simulink model "Complete_ballsegway_model"  (R2024b)
settings: Solver=VariableStepAuto  StartTime=0.0  StopTime=10  RelTol=1e-3
settings Model: Creator=sumit  LastModifiedBy=yugan
settings DebuggingCC: AlgebraicLoopMsg=none

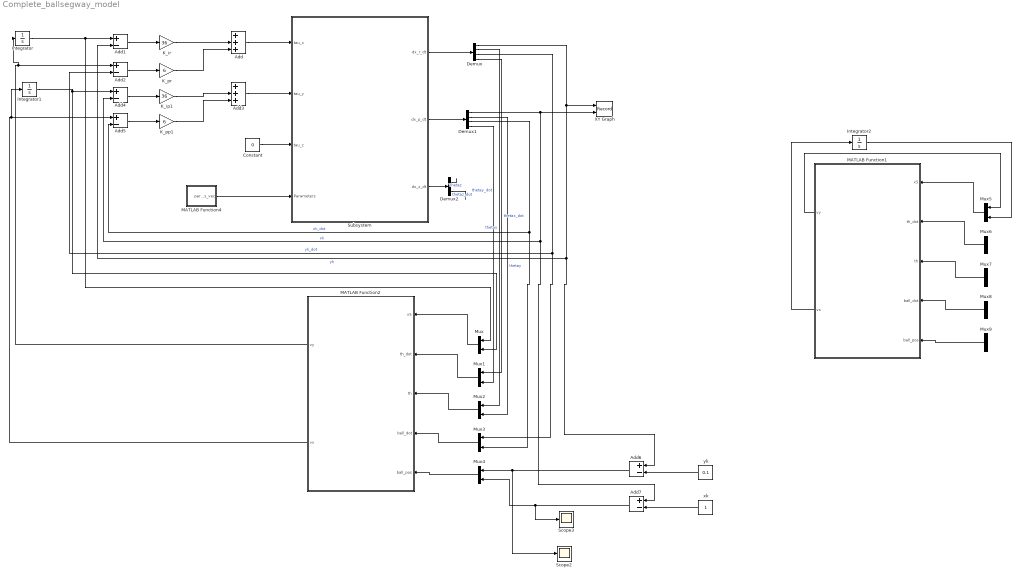
== system Complete_ballsegway_model ==
  Add : Sum  Inputs=+++
  Add{1..2,4..7} (6 alike) : Sum  Inputs=+-
  Add3 : Sum  Inputs=+++
  Constant : Constant  Value=0
  Demux : Demux
  Demux1 : Demux
  Demux2 : Demux  Outputs=2
  Integrator : Integrator
  Integrator1 : Integrator
  Integrator2 : Integrator
  K_ip1 : Gain  Gain=36
  K_ir : Gain  Gain=36
  K_pp1 : Gain  Gain=6
  K_pr : Gain  Gain=6
  MATLAB Function1 : MATLAB Function  TreatAsAtomicUnit=on
  MATLAB Function2 : MATLAB Function  TreatAsAtomicUnit=on
  MATLAB Function4 : MATLAB Function  TreatAsAtomicUnit=on
  Mux{,1..9} (10 alike) : Mux  Inputs=2
  Scope2 : Scope
  Scope3 : Scope
  Subsystem : Subsystem
  XY Graph : Record  FileSettingsInternal="{\"entries\":[{\"content\":{\"excelSettings\":{\"content\":{},\"type\":\"Streamout.ExcelSettings\"}},\"type\":\"Streamout.FileSettingStorage\",\"uuid\":\"\"}],\"packageUris\":[\"http:\\/\\/schema.mathworks.com\\/mf0\\/streamout_blocks\\/R2020a\"],\"version\":\"1.0\"}"  Layout=[1 1]  SignalsInternal="{\"entries\":[{\"content\":{\"signals\":[{\"content\":{\"blockPath\":[],\"dimensions\":[1,1],\"domain\":\"\",\"lineColor\":\"#a2142f\",\"plots\":[ 1 ],\"port\":1,\"signalID\":1,\"signalName\":\"yk\"},\"type\":\"RecordBlkView.Signal\",\"uuid\":\"\"},{\"content\":{\"blockPath\":[],\"dimensions\":[1,1],\"domain\":\"\",\"lineColor\":\"#139fff\",\"plots\":[ 1 ],\"port\":2,\"signalID\":2,\"signalName\":\"xk\"},\"type\":\"RecordBlkView.Signal\",\"uuid\":\"\"}]},\"type\":\"RecordBlkView.InputSignals\",\"uuid\":\"\"}],\"packageUris\":[\"http:\\/\\/schema.mathworks.com\\/mf0\\/streamout_blocks\\/R2020a\"],\"version\":\"1.0\"}"  VisualizationBindings="{\"xyplotplugin\":{\"info\":[{\"series\":[{\"bindingParametersList\":[{\"parameter\":\"Y-Axis\",\"signalID\":1,\"signalName\":\"yk\"}],\"seriesID\":0}],\"subplotID\":1}]}}"  CompatibilityTag=XY
  xk : Constant
  yk : Constant  Value=0.1
  wires:
  Subsystem/3(dx_z_dt) -> Demux2/1
  MATLAB Function4/1(params_vec) -> Subsystem/4(Parameters)
  Mux/1 -> MATLAB Function2/1(x5)
  Integrator1/1 -> Mux/2, Add4/1
  Add/1 -> Subsystem/1(tau_x)
  K_ir/1 -> Add/2
  Add1/1 -> K_ir/1
  Subsystem/1(dx_r_dt) -> Demux/1
  Subsystem/2(dx_p_dt) -> Demux1/1
  Demux/1 -> Add1/2, Add6/1, XY Graph/1  "yk"
  Demux/2 -> Mux2/1  "thetax"
  Demux/3 -> Mux3/1, Add2/2  "yk_dot"
  Demux/4 -> Mux1/1  "thetax_dot"
  Demux1/2 -> Mux2/2  "thetay"
  Demux1/3 -> Mux3/2, Add5/2  "xk_dot"
  Demux1/4 -> Mux1/2  "thetay_dot"
  Demux2/1 -> ?  "Thetaz"
  Demux2/2 -> ?  "thetaz_dot"
  Integrator/1 -> Mux/1, Add1/1
  K_pr/1 -> Add/3
  Add2/1 -> K_pr/1
  Demux1/1 -> Add7/1, Add4/2, XY Graph/2  "xk"
  Add4/1 -> K_ip1/1
  K_pp1/1 -> Add3/3
  K_ip1/1 -> Add3/2
  Add3/1 -> Subsystem/2(tau_y)
  Add5/1 -> K_pp1/1
  Constant/1 -> Subsystem/3(tau_z)
  Mux1/1 -> MATLAB Function2/2(th_dot)
  Mux2/1 -> MATLAB Function2/3(th)
  Mux3/1 -> MATLAB Function2/4(ball_dot)
  Mux4/1 -> MATLAB Function2/5(ball_pos)
  Add6/1 -> Scope2/1, Mux4/1
  yk/1 -> Add6/2
  Add7/1 -> Scope3/1, Mux4/2
  xk/1 -> Add7/2
  MATLAB Function2/1(vy) -> Add2/1, Integrator/1
  MATLAB Function2/2(vx) -> Add5/1, Integrator1/1
  MATLAB Function1/1(vy) -> Mux5/1
  Mux5/1 -> MATLAB Function1/1(x5)
  Mux7/1 -> MATLAB Function1/3(th)
  Mux8/1 -> MATLAB Function1/4(ball_dot)
  Mux6/1 -> MATLAB Function1/2(th_dot)
  Mux9/1 -> MATLAB Function1/5(ball_pos)
  MATLAB Function1/2(vx) -> Integrator2/1
  ? -> Mux6/1
  ? -> Mux6/2
  ? -> Mux7/1
  ? -> Mux7/2
  ? -> Mux8/1
  ? -> Mux8/2
  ? -> Mux9/1
  ? -> Mux9/2
  Integrator2/1 -> Mux5/2

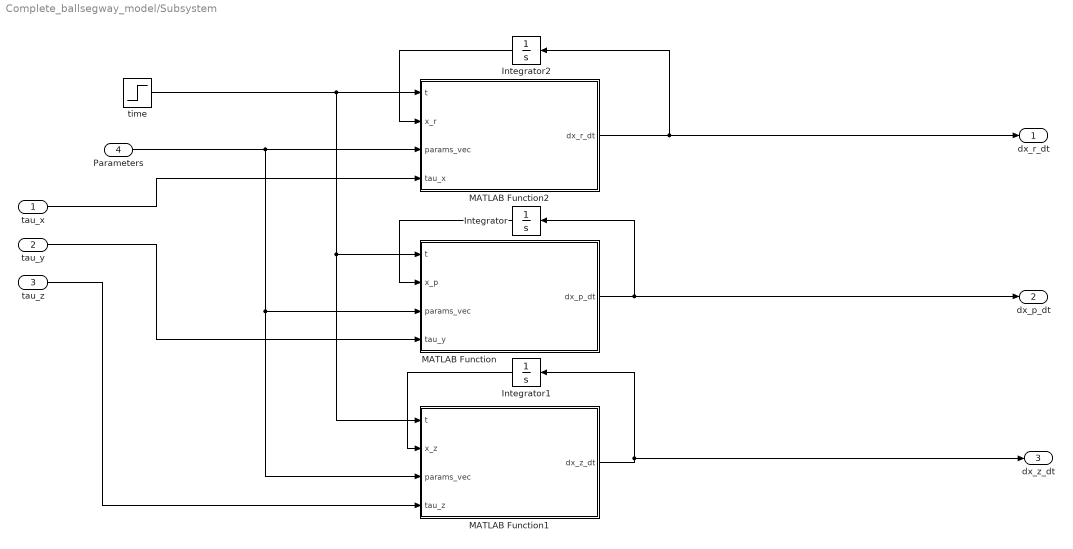
== system Complete_ballsegway_model/Subsystem ==
  tau_x : Inport
  tau_y : Inport  Port=2
  tau_z : Inport  Port=3
  Parameters : Inport  Port=4
  Integrator : Integrator  InitialCondition=[0; 0; 0; 0]
  Integrator1 : Integrator  InitialCondition=[0 ;0]
  Integrator2 : Integrator  InitialCondition=[0; 0; 0; 0]
  MATLAB Function : MATLAB Function  TreatAsAtomicUnit=on
  MATLAB Function1 : MATLAB Function  TreatAsAtomicUnit=on
  MATLAB Function2 : MATLAB Function  TreatAsAtomicUnit=on
  time : Step  After=10  SampleTime=0
  dx_r_dt : Outport
  dx_p_dt : Outport  Port=2
  dx_z_dt : Outport  Port=3
  wires:
  time/1 -> MATLAB Function1/1(t), MATLAB Function/1(t), MATLAB Function2/1(t)
  Integrator1/1 -> MATLAB Function1/2(x_z)
  Parameters/1 -> MATLAB Function/3(params_vec), MATLAB Function1/3(params_vec), MATLAB Function2/3(params_vec)
  Integrator2/1 -> MATLAB Function2/2(x_r)
  MATLAB Function1/1(dx_z_dt) -> Integrator1/1, dx_z_dt/1
  tau_z/1 -> MATLAB Function1/4(tau_z)
  Integrator/1 -> MATLAB Function/2(x_p)
  tau_y/1 -> MATLAB Function/4(tau_y)
  tau_x/1 -> MATLAB Function2/4(tau_x)
  MATLAB Function/1(dx_p_dt) -> Integrator/1, dx_p_dt/1
  MATLAB Function2/1(dx_r_dt) -> dx_r_dt/1, Integrator2/1

== matlab function Complete_ballsegway_model/Subsystem/MATLAB Function1 ==
  data: t input; dx_z_dt output; x_z input; params_vec input; tau_z input
function dx_z_dt = yaw_dynamics(t, x_z, params_vec, tau_z)
% yaw_dynamics.m
%
% 1-DOF yaw dynamic model for Ball Segway.
%
% State x_z = [theta_z ; theta_z_dot]
% params_vec = 20×1 numeric parameter vector (from init_params)
% Output dx_z_dt = state derivative (2×1)

%% ---------------------------------------------------------
% Unpack Parameters From Vector
%% ---------------------------------------------------------

mk  = params_vec(1);     %#ok<NASGU> (not used)
Ik  = params_vec(2);
ma  = params_vec(3);     %#ok<NASGU>
Ix  = params_vec(4);     %#ok<NASGU>
Iy  = params_vec(5);
Iz  = params_vec(6);
l   = params_vec(7);     %#ok<NASGU>
alpha_rad = params_vec(8);
rk  = params_vec(9);
rw  = params_vec(10);
bx  = params_vec(11);    %#ok<NASGU>
dx  = params_vec(12);    %#ok<NASGU>
by  = params_vec(13);    %#ok<NASGU>
dy  = params_vec(14);    %#ok<NASGU>
bry = params_vec(15);    %#ok<NASGU>
dry = params_vec(16);    %#ok<NASGU>
brx = params_vec(17);    %#ok<NASGU>
drx = params_vec(18);    %#ok<NASGU>
g   = params_vec(19);    %#ok<NASGU>
k_motor = params_vec(20); %#ok<NASGU>

% Keep notation same as your original code
I_k_param = Ik;
I_w = Iy;


%% ---------------------------------------------------------
% Extract States
%% ---------------------------------------------------------

theta_z     = x_z(1);
theta_z_dot = x_z(2);


%% ---------------------------------------------------------
% Yaw Dynamics (Eq. 13)
%% ---------------------------------------------------------

num = I_k_param * (rk / rw) * tau_z;

den = I_k_param * Iz + ...
      3 * (I_k_param + Iz) * I_w * (rk / rw)^2 * sin(alpha_rad)^2;

theta_z_ddot = num / den;


%% ---------------------------------------------------------
% Return Derivative
%% ---------------------------------------------------------

dx_z_dt = [ theta_z_dot ;
            theta_z_ddot ];

end

== matlab function Complete_ballsegway_model/Subsystem/MATLAB Function ==
  data: t input; dx_p_dt output; x_p input; params_vec input; tau_y input
function dx_p_dt = pitch_dynamics(t, x_p, params_vec, tau_y)
% pitch_dynamics.m
%
% 2-DOF dynamic model in the X–Z plane (pitch plane).
%
% State x_p = [x_k ; theta_y ; x_k_dot ; theta_y_dot]
% params_vec = 20×1 vector from init_params()
% Output dx_p_dt = state derivative (4×1)

%% ---------------------------------------------------------
% Unpack Parameters from Vector
%% ---------------------------------------------------------

mk  = params_vec(1);     % ball mass
Ik  = params_vec(2);     % ball inertia
ma  = params_vec(3);     % body mass
Ix  = params_vec(4);     % inertia about x
Iy  = params_vec(5);     % inertia about y
Iz  = params_vec(6);     % inertia about z
l   = params_vec(7);     % COM height
alpha_rad = params_vec(8); % zenith angle
rk  = params_vec(9);     % ball radius
rw  = params_vec(10);    % omniwheel radius
bx  = params_vec(11);
dx  = params_vec(12);
by  = params_vec(13);
dy  = params_vec(14);
bry = params_vec(15);
dry = params_vec(16);
brx = params_vec(17);
drx = params_vec(18);
g   = params_vec(19);    % gravity
k_motor = params_vec(20);

% Keep original notation
I_k_param = Ik;
I_w = Iy;    % consistent with roll dynamics formulation


%% ---------------------------------------------------------
% Extract State Variables
%% ---------------------------------------------------------

x_k         = x_p(1);
theta_y     = x_p(2);
x_k_dot     = x_p(3);
theta_y_dot = x_p(4);

q_y_dot = [x_k_dot ; theta_y_dot];


%% ---------------------------------------------------------
% Mass Matrix M(q)   (Eq. 8)
%% ---------------------------------------------------------

M11 = mk + (I_k_param / rk^2) + ma + ...
      (3*I_w*cos(alpha_rad)^2) / (2*rw^2);

M12 =   ma*l*cos(theta_y) ...
      - (3*I_w*cos(alpha_rad)^2)/(2*rw^2) * rk;

M21 = M12;

M22 = ma*l^2 + ...
      (3*I_w*rk^2*cos(alpha_rad)^2)/(2*rw^2) + Iy;

M_y = [M11 M12; M21 M22];


%% ---------------------------------------------------------
% Coriolis–Centrifugal Vector
%% ---------------------------------------------------------

C_y = [ 0                            -ma*l*theta_y_dot*sin(theta_y);
        0                             0 ];


%% ---------------------------------------------------------
% Gravity Vector
%% ---------------------------------------------------------

G_y = [0;
       -ma*g*l*sin(theta_y)];


%% ---------------------------------------------------------
% Friction Vector (ignored)
%% ---------------------------------------------------------

D_y = [0; 0];


%% ---------------------------------------------------------
% Input Torque Vector
%% ---------------------------------------------------------

Q_y = [ -(1/rw) * tau_y ;
         (rk/rw) * tau_y ];


%% ---------------------------------------------------------
% Solve q¨ = M⁻¹ (Q – C q̇ – D – G)
%% ---------------------------------------------------------

q_y_ddot = M_y \ (Q_y - C_y*q_y_dot - D_y - G_y);


%% ---------------------------------------------------------
% Output State Derivatives
%% ---------------------------------------------------------

dx_p_dt = [ x_k_dot ;
            theta_y_dot ;
            q_y_ddot(1) ;
            q_y_ddot(2) ];

end

== matlab function Complete_ballsegway_model/Subsystem/MATLAB Function2 ==
  data: t input; dx_r_dt output; x_r input; params_vec input; tau_x input
function dx_r_dt = roll_dynamics(t, x_r, params_vec, tau_x)
% roll_dynamics.m
%
% State vector x_r = [y_k, theta_x, y_k_dot, theta_x_dot]'

%% 1. Unpack State
y_k         = x_r(1);
theta_x     = x_r(2);
y_k_dot     = x_r(3);
theta_x_dot = x_r(4);
q_x_dot     = [y_k_dot; theta_x_dot];

%% 2. Unpack parameters from vector
mk  = params_vec(1);
Ik  = params_vec(2);
ma  = params_vec(3);
Ix  = params_vec(4);
Iy  = params_vec(5);
Iz  = params_vec(6);
l   = params_vec(7);
alpha_rad = params_vec(8);
rk  = params_vec(9);
rw  = params_vec(10);
bx  = params_vec(11);
dx  = params_vec(12);
by  = params_vec(13);   % USED
dy  = params_vec(14);   % USED
bry = params_vec(15);
dry = params_vec(16);
brx = params_vec(17);   % USED
drx = params_vec(18);   % USED
g   = params_vec(19);
k_motor = params_vec(20);

%% 3. Dynamics Matrices

% Mass Matrix
M11 = mk + (Ik / rk^2) + ma + (3*Iy*cos(alpha_rad)^2)/(2*rw^2);
M12 = (3*Iy*cos(alpha_rad)^2)/(2*rw^2)*rk - ma*l*cos(theta_x);
M21 = M12;
M22 = ma*l^2 + (3*Iy*rk^2*cos(alpha_rad)^2)/(2*rw^2) + Ix;
M_x = [M11 M12; M21 M22];

% Coriolis Matrix
C_x = [ 0                     ma*l*theta_x_dot*sin(theta_x);
        0                     0 ];

% Gravity Vector
G_x = [ 0 ;
       -ma*g*l*sin(theta_x) ];

%% 4. Friction / Damping Vector (NEW)
% D(q̇) = [by*y_k_dot + dy*sign(y_k_dot) ;
%         brx*theta_x_dot + drx*sign(theta_x_dot)]

D1 = by * y_k_dot     + dy  * sign(y_k_dot);
D2 = brx * theta_x_dot + drx * sign(theta_x_dot);
D_x = [D1 ; D2];

%% 5. Control torque vector
Q_x = [ (1/rw)*tau_x ;
         (rk/rw)*tau_x ];

%% 6. Compute accelerations
q_x_ddot = M_x \ (Q_x - C_x*q_x_dot - D_x - G_x);

%% 7. Output derivative
dx_r_dt = [
    y_k_dot ;
    theta_x_dot ;
    q_x_ddot(1) ;
    q_x_ddot(2)
];

end

== matlab function Complete_ballsegway_model/MATLAB Function1 ==
  data: x5 input; th_dot input; th input; ball_dot input; ball_pos input; vy output size=[1]; vx output size=[1]
function [vy, vx] = LQR_Block(x5, th_dot, th, ball_dot, ball_pos)
%(x5, th, th_dot, )
% ========================================================================
%   REAL-TIME LQR CONTROLLER BLOCK
%   Applies pre-calculated gains Kr and Kp to the system states.
%
%   This block EXPECTS 'Kr' and 'Kp' to be passed in as parameters.
% ========================================================================

%% ------------------------------------------------------------
% BUILD STATE VECTORS
% **FIXED**: Swapped states back. Roll (y/2) and Pitch (x/1)
%            Please verify th(1) vs th(2) matches your setup.
%            Commonly: th(1)=pitch, th(2)=roll
%% ------------------------------------------------------------

Kr = [-6.98, 4.45, 20.88, 6.09, 5.11];  % example row
Kp = [-3.27, 4.01, 29.07, 8.54, 5.72];  % example row


xr = [ th(1);         % Roll angle
       th_dot(1);     % Roll rate
       ball_pos(1);   % Ball X position (relative to roll)
       ball_dot(1);   % Ball X velocity
       x5(1)          % Roll integral term
       ];
       
xp = [ th(2);         % Pitch angle
       th_dot(2);     % Pitch rate
       ball_pos(2);   % Ball Y position (relative to pitch)
       ball_dot(2);   % Ball Y velocity
       x5(2)          % Pitch integral term
       ];

%% ------------------------------------------------------------
% CONTROL LAWS (Simple multiplication)
%% ------------------------------------------------------------
vy = -Kr * xr;   % Roll command
vx = -Kp * xp;   % Pitch command
end

== matlab function Complete_ballsegway_model/MATLAB Function4 ==
  data: params_vec output size=[20 1]
function params_vec = init_params()
% init_params.m
% Returns parameters as a 20×1 vector (NO STRUCT)

mk  = 19.6;                   % (1) ball mass
Ik  = 0.38;                   % (2) ball inertia
ma  = 68;                     % (3) body mass
Ix  = 12.1;                   % (4) body inertia x
Iy  = 11.67;                  % (5) body inertia y
Iz  = 1.08;                   % (6) body inertia z
l   = 0.38;                   % (7) COM height
a   = deg2rad(65.5);          % (8) zenith angle
rk  = 0.22;                   % (9) ball radius
rw  = 0.10;                   % (10) omniwheel radius
bx  = 0.10;                   % (11) viscous friction xz
dx  = 0.01;                   % (12) coulomb friction xz
by  = 0.10;                   % (13) viscous friction yz
dy  = 0.01;                   % (14) coulomb friction yz
bry = 0.12;                   % (15) body/ball viscous xz
dry = 0.02;                   % (16) coulomb xz
brx = 0.12;                   % (17) body/ball viscous yz
drx = 0.02;                   % (18) coulomb yz
g   = 9.81;                   % (19) gravity
k_motor = 1;                  % (20) motor constant


% Return as vector
params_vec = [
    mk; Ik; ma; Ix; Iy; Iz;
    l; a; rk; rw;
    bx; dx; by; dy;
    bry; dry; brx; drx;
    g; k_motor
];
end

== matlab function Complete_ballsegway_model/MATLAB Function2 ==
  data: x5 input; th_dot input; th input; ball_dot input; ball_pos input; vy output size=[1]; vx output size=[1]
function [vy, vx] = LQR_Block(x5, th_dot, th, ball_dot, ball_pos)
%(x5, th, th_dot, )
% ========================================================================
%   REAL-TIME LQR CONTROLLER BLOCK
%   Applies pre-calculated gains Kr and Kp to the system states.
%
%   This block EXPECTS 'Kr' and 'Kp' to be passed in as parameters.
% ========================================================================

%% ------------------------------------------------------------
% BUILD STATE VECTORS
% **FIXED**: Swapped states back. Roll (y/2) and Pitch (x/1)
%            Please verify th(1) vs th(2) matches your setup.
%            Commonly: th(1)=pitch, th(2)=roll
%% ------------------------------------------------------------

Kr = [-6.98, 4.45, 20.88, 6.09, 5.11];  % example row
Kp = [-3.27, 4.01, 29.07, 8.54, 5.72];  % example row


xr = [ th(1);         % Roll angle
       th_dot(1);     % Roll rate
       ball_pos(1);   % Ball X position (relative to roll)
       ball_dot(1);   % Ball X velocity
       x5(1)          % Roll integral term
       ];
       
xp = [ th(2);         % Pitch angle
       th_dot(2);     % Pitch rate
       ball_pos(2);   % Ball Y position (relative to pitch)
       ball_dot(2);   % Ball Y velocity
       x5(2)          % Pitch integral term
       ];

%% ------------------------------------------------------------
% CONTROL LAWS (Simple multiplication)
%% ------------------------------------------------------------
vy = -Kr * xr;   % Roll command
vx = -Kp * xp;   % Pitch command
end
